simulink model "chap7_14sim"  (Simulink 5.0)
settings: Solver=ode45  StartTime=0.0  StopTime=15.0  RelTol=1e-3
settings Model: LastModifiedBy=Administrator

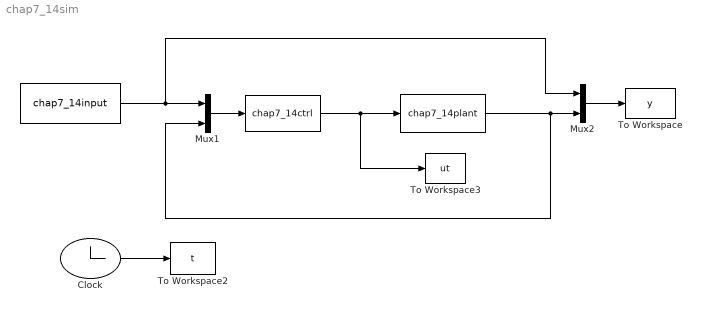
== system chap7_14sim ==
  "  " : S-Function  FunctionName=chap7_14plant
  "   " : S-Function  FunctionName=chap7_14input
  "    " : S-Function  FunctionName=chap7_14ctrl
  Clock : Clock
      settings: Decimation=10
  Mux1 : Mux  Inputs=2
  Mux2 : Mux  Inputs=2
  To Workspace : ToWorkspace  VariableName=y  SampleTime=-1  SaveFormat=Array
  To Workspace2 : ToWorkspace  VariableName=t  SampleTime=-1  SaveFormat=Array
  To Workspace3 : ToWorkspace  VariableName=ut  SampleTime=-1  SaveFormat=Array
  wires:
  "  "/1 -> Mux2/2, Mux1/2
  "    "/1 -> To Workspace3/1, "  "/1
  Clock/1 -> To Workspace2/1
  Mux1/1 -> "    "/1
  "   "/1 -> Mux2/1, Mux1/1
  Mux2/1 -> To Workspace/1
